simulink model "xuanzuo"  (R2022a)
settings: Solver=VariableStepAuto  StartTime=0.0  StopTime=10.0  RelTol=1e-3
libraries: dspswit3 x2
settings Model: Creator=惠普  LastModifiedBy=惠普

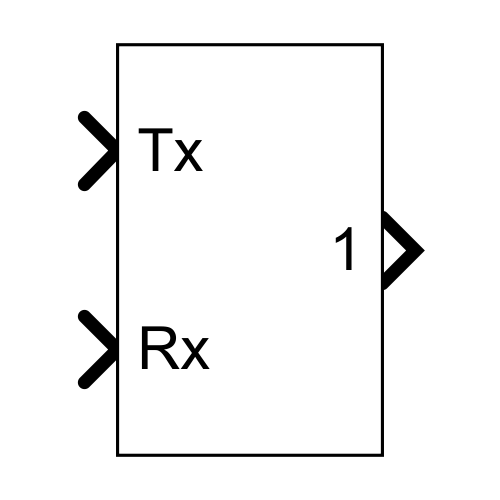
[thumbnail: Simulink's stored preview of the top-level diagram]
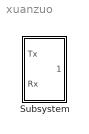
== system xuanzuo ==
  Subsystem : Subsystem

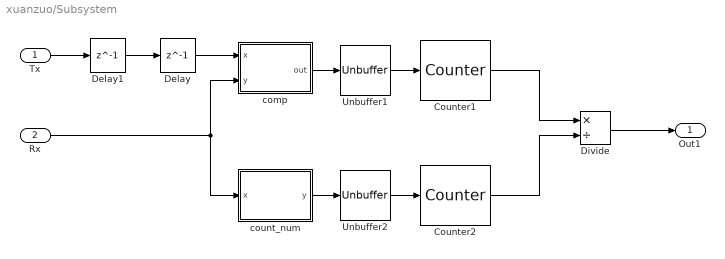
== system xuanzuo/Subsystem ==
  Tx : Inport
  Rx : Inport  Port=2
  Counter1 : dspswit3/Counter  Direction=Up  CountEvent=Rising edge  CounterSize=User defined  MaxCount=1000000  InitialCount=0  Output=Count  HitValue=32  ResetInput=off  SamplesPerFrame=1  Ts=1  CntDtype=double  HitDtype=Logical
  Counter2 : dspswit3/Counter  Direction=Up  CountEvent=Rising edge  CounterSize=User defined  MaxCount=1000000  InitialCount=0  Output=Count  HitValue=32  ResetInput=off  SamplesPerFrame=1  Ts=1  CntDtype=double  HitDtype=Logical
  Delay : Delay  DelayLength=1  InitialCondition=0
  Delay1 : Delay  DelayLength=1  InitialCondition=0
  Divide : Product  Inputs=*/
  Unbuffer1 : Unbuffer
  Unbuffer2 : Unbuffer
  comp : MATLAB Function  TreatAsAtomicUnit=on
  count_num : MATLAB Function  TreatAsAtomicUnit=on
  Out1 : Outport
  wires:
  Delay1/1 -> Delay/1
  Delay/1 -> comp/1(x)
  Divide/1 -> Out1/1
  Counter1/1 -> Divide/1
  Unbuffer1/1 -> Counter1/1
  count_num/1(y) -> Unbuffer2/1
  Rx/1 -> count_num/1(x), comp/2(y)
  comp/1(out) -> Unbuffer1/1
  Tx/1 -> Delay1/1
  Counter2/1 -> Divide/2
  Unbuffer2/1 -> Counter2/1

== matlab function xuanzuo/Subsystem/count_num ==
  data: x input; y output
function y = count_num(x)
len = length(x);
y = zeros(len,1);
y(1,1) = 1;
return

== matlab function xuanzuo/Subsystem/comp ==
  data: x input; out output; y input
function out = comp(x,y)
len = length(x);
out = zeros(len,1);
for p = 1:len
    if (x(p) ~= y(p))
        out(1,1) = 1;
        return
    end
end
return
